simulink library "lib_transmission2"  (Simulink 10.1)
settings: Solver=VariableStepAuto  StartTime=0.0  StopTime=10.0  RelTol=1e-3
undefined symbols (not defined in the file or in its folder): cyc_mph, fc_map_spd, fc_max_trq, fc_spd_scale, fc_trq_scale, fd_inertia, fd_loss, fd_ratio, gb_gear_number_lookup, gb_gears_num, gb_inertia, gb_loss_const, gb_loss_input_spd_coeff, gb_loss_input_trq_coeff, gb_loss_output_spd_coeff, gb_loss_output_trq_coeff, gb_num_init, gb_ratio, gb_shift_delay, gb_spd_scale, gb_trq_scale, htc_inertia, htc_k_adv, htc_k_adv_coast, htc_lockup, htc_lockup_load, htc_lockup_spd, htc_lu_gear_range, htc_max_coast_tr, htc_min_coast_tr, htc_pump_loss_spd, htc_pump_loss_trq_lockup, htc_pump_loss_trq_unlock, htc_sr, htc_sr_coast, htc_tr, htc_tr_coast, htc_unlock_spd, mc_map_spd, mc_max_trq, mc_overtrq_factor, mc_spd_scale, mc_trq_scale, tc_loss, tc_mc_to_fc_ratio, tx_eff_map, tx_map_spd, tx_map_trq, tx_pg_r, tx_pg_s, tx_speed_dep, vc_clutch_bool, vc_idle_spd, vc_launch_spd, wh_radius
undefined symbols (not defined in the file): gb_dnshift_load, gb_dnshift_spd, gb_map_spd_out, gb_map_trq_in, gb_map_trq_out, gb_upshift_load, gb_upshift_spd, logFlag
libraries: lib_controls x1, lib_etc x1, lib_controls2 x1, lib_transmission x1
(part 13 of 17)

== system lib_transmission2/gearbox <gb>/gearbox model & interface/gearbox model/gearbox controller interface ==
  T_gb_out : Inport
  w_gb_out : Inport  Port=2
  eta_gb : Inport  Port=3
  enhancedToWorkspace1 : Subsystem  mask(enhancedToWorkspace){generalName=generalName, specificName=gear_ratio, logFlag=logFlag}
      mask prompts: generalName "General Name [char-evaluated]"; specificName "Specific Name [char-literal]"; logFlag "Enable flag (1=on,0=off)"
      mask help: A wrapper for the Simulink "To Workspace" block that allows you to evaluate the name of the variable to log to workspace. This is useful to avoid the double logging errors that occur when you pull in two library models that attempt to log to the same variable.
      mask init:
      | enhancedToWsMaker
      settings: CopyFcn=breakLinkCopyFcn  ParentCloseFcn=breakLinkParCloseFcn
      mask Help:
      | <h2>Enhanced To Workspace Block</h2>
      | <h3>Parameters</h3>
      | <UL>
      | <li><b>General Name:</b> This is the more general name of the variable. Variables are saved to the workspace as <i>generalName_specificName</i>. Note that this is an evaluated variable. If you would like to type in the value directly, it must be surrounded with single quotes. Otherwise you can input the name of a variable containing a char string.</li>
      | <li><b>Specific Name:</b> This is the specific name of the variable. Note that this is input as a char literal (i.e., you don't need quotes).</li>
      | <li><b>Enable Flag:</b> This flag should have the value of 0 or 1. If 0, the variable will not be logged to the workspace. If 1, the variable will be logged. This is done so that variable logging can be turned off to improve speed.</li>
      | </ul>
      | <h3>Overview</h3>
      | <p>The enhanced to workspace block was put together to allow one to dynamically resolve variable names at run time in simulink. This is most powerful when used in conjunction with a masked subsystem to allow multiple instances of that masked subsytem to be used in the same model. The strategy is to set the generalName in the block mask which will allow the block to change the general name for all variable logging on the fly.
      | <h3>Helper Files</h3>
      | <p>Three m-files are required by the enhancedToWorkspace block. These files are located in the &lt; ADVISOR root &gt;/GUI directory :
      | <ul>
      | <li><i>enhancedToWsMaker.m</i> This file runs the mask initialization for the block</li>
      | <li><i>breakLinkCopyFcn.m</i> This file is used by the block callback when the simulink block is copied. It is necessary to break the link to the enhancedToWorkspace similar to the To Workspace block in order for it to be able to configure itself. (Try copying simulink's To Workspace block--it is impossible to make a link)</li>
      | <li><i>breakLinkParCloseFcn.m</i> This file is similar to the breakLinkCopyFcn and is used when a parent system is closed</li>
      | </ul>
      | <hr>
      | 
      | <p>Created 2003-Jan-21, Michael Patrick O'Keefe, NREL</p>
      mask Display: disp([generalName,'_',specificName])
  enhancedToWorkspace8 : Subsystem  mask(enhancedToWorkspace){generalName=generalName, specificName=shifting, logFlag=logFlag}
      mask prompts: generalName "General Name [char-evaluated]"; specificName "Specific Name [char-literal]"; logFlag "Enable flag (1=on,0=off)"
      mask help: A wrapper for the Simulink "To Workspace" block that allows you to evaluate the name of the variable to log to workspace. This is useful to avoid the double logging errors that occur when you pull in two library models that attempt to log to the same variable.
      mask init:
      | enhancedToWsMaker
      settings: CopyFcn=breakLinkCopyFcn  ParentCloseFcn=breakLinkParCloseFcn
      mask Help:
      | <h2>Enhanced To Workspace Block</h2>
      | <h3>Parameters</h3>
      | <UL>
      | <li><b>General Name:</b> This is the more general name of the variable. Variables are saved to the workspace as <i>generalName_specificName</i>. Note that this is an evaluated variable. If you would like to type in the value directly, it must be surrounded with single quotes. Otherwise you can input the name of a variable containing a char string.</li>
      | <li><b>Specific Name:</b> This is the specific name of the variable. Note that this is input as a char literal (i.e., you don't need quotes).</li>
      | <li><b>Enable Flag:</b> This flag should have the value of 0 or 1. If 0, the variable will not be logged to the workspace. If 1, the variable will be logged. This is done so that variable logging can be turned off to improve speed.</li>
      | </ul>
      | <h3>Overview</h3>
      | <p>The enhanced to workspace block was put together to allow one to dynamically resolve variable names at run time in simulink. This is most powerful when used in conjunction with a masked subsystem to allow multiple instances of that masked subsytem to be used in the same model. The strategy is to set the generalName in the block mask which will allow the block to change the general name for all variable logging on the fly.
      | <h3>Helper Files</h3>
      | <p>Three m-files are required by the enhancedToWorkspace block. These files are located in the &lt; ADVISOR root &gt;/GUI directory :
      | <ul>
      | <li><i>enhancedToWsMaker.m</i> This file runs the mask initialization for the block</li>
      | <li><i>breakLinkCopyFcn.m</i> This file is used by the block callback when the simulink block is copied. It is necessary to break the link to the enhancedToWorkspace similar to the To Workspace block in order for it to be able to configure itself. (Try copying simulink's To Workspace block--it is impossible to make a link)</li>
      | <li><i>breakLinkParCloseFcn.m</i> This file is similar to the breakLinkCopyFcn and is used when a parent system is closed</li>
      | </ul>
      | <hr>
      | 
      | <p>Created 2003-Jan-21, Michael Patrick O'Keefe, NREL</p>
      mask Display: disp([generalName,'_',specificName])
  gear_ratio : Outport  InitialOutput=0
  shifting : Outport  Port=2  InitialOutput=0
  tag scope: T_gb_out=scoped, eta_gb=scoped, w_gb_out=scoped
  wires:
  [gear_ratio] -> gear_ratio/1, enhancedToWorkspace1/1(In1)
  eta_gb/1 -> [eta_gb]
  w_gb_out/1 -> [w_gb_out]
  T_gb_out/1 -> [T_gb_out]
  [shifting] -> shifting/1, enhancedToWorkspace8/1(In1)

== system lib_transmission2/gearbox <gb>/gearbox model & interface/gearbox model/gearing (Nm) (rad/s) ==
  "output shaft torque and speed  (Nm), (rad/s)" : Inport
  gear ratio : Inport  Port=2
  Demux : Demux  Outputs=2
  Fcn1 : Fcn  Expr=1/u
  Product2 : Product  SaturateOnIntegerOverflow=on
  Product3 : Product  SaturateOnIntegerOverflow=on
  input shaft torque (Nm) : Outport  InitialOutput=0
  input shaft speed (rad/s) : Outport  Port=2  InitialOutput=0
  wires:
  Product3/1 -> input shaft speed (rad/s)/1
  Product2/1 -> input shaft torque (Nm)/1
  Fcn1/1 -> Product2/2
  "output shaft torque and speed  (Nm), (rad/s)"/1 -> Demux/1
  gear ratio/1 -> Fcn1/1, Product3/2
  Demux/1 -> Product2/1
  Demux/2 -> Product3/1

== system lib_transmission2/gearbox <gb>/gearbox model & interface/gearbox model/gearing (Nm) (rad/s)1 ==
  input shaft torque (Nm) : Inport
  input shaft speed (rad/s) : Inport  Port=2
  gear ratio : Inport  Port=3
  Fcn1 : Fcn  Expr=1/u
  Product2 : Product  SaturateOnIntegerOverflow=on
  Product3 : Product  SaturateOnIntegerOverflow=on
  output shaft torque (Nm) : Outport  InitialOutput=0
  output shaft speed (rad/s) : Outport  Port=2  InitialOutput=0
  wires:
  Fcn1/1 -> Product3/1
  gear ratio/1 -> Product2/2, Fcn1/1
  Product3/1 -> output shaft speed (rad/s)/1
  Product2/1 -> output shaft torque (Nm)/1
  input shaft torque (Nm)/1 -> Product2/1
  input shaft speed (rad/s)/1 -> Product3/2

== system lib_transmission2/gearbox <gb>/gearbox model & interface/gearbox model/help ==

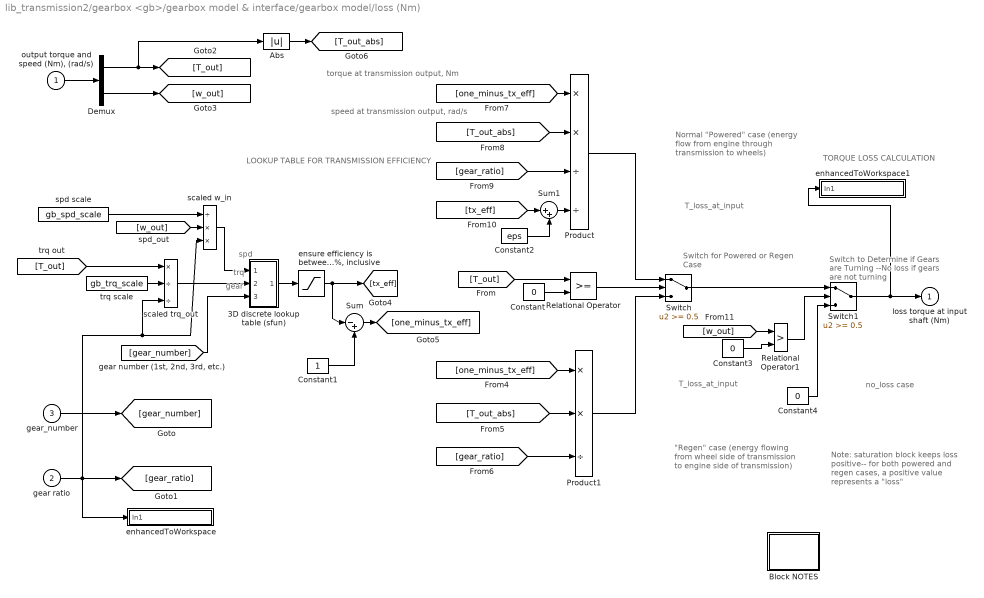
== system lib_transmission2/gearbox <gb>/gearbox model & interface/gearbox model/loss (Nm) ==
  note: TORQUE LOSS CALCULATION
  note: gear
  note: trq
  note: spd
  note: torque at transmission output, Nm
  note: speed at transmission output, rad/s
  note: no_loss case
  note: Note: saturation block keeps
      | loss positive-- for both powered
      | and regen cases, a
      | positive value represents a "loss"
  note: Switch for Powered
      |  or Regen Case
  note: Switch to Determine
      | if Gears are Turning
      | --No loss if gears
      | are not turning
  note: Normal "Powered" case
      | (energy flow from engine
      | through transmission to wheels)
  note: T_loss_at_input
  note: "Regen" case
      | (energy flowing from
      | wheel side of transmission
      | to engine side of transmission)
  note: T_loss_at_input
  note: LOOKUP TABLE FOR TRANSMISSION EFFICIENCY
  "output torque and speed (Nm), (rad/s)" : Inport
  gear ratio : Inport  Port=2
  gear_number : Inport  Port=3
  3D discrete lookup table (sfun) : Subsystem  AncestorBlock=|  mask{tx_map_spd=tx_map_spd, tx_map_trq=tx_map_trq, tx_eff_map=tx_eff_map}
      | lib_transmission/SubLibraries/3D discrete lookup
      | table (sfun)
      mask prompts: tx_map_spd "Row Lookup"; tx_map_trq "Column Lookup"; tx_eff_map "Lookup Matrix"
  Abs : Abs  SaturateOnIntegerOverflow=on
  Block NOTES : Subsystem
      mask Display: disp('Block\nNOTES')
  Constant : Constant  Value=0
  Constant1 : Constant
  Constant2 : Constant  Value=eps
  Constant3 : Constant  Value=0
  Constant4 : Constant  Value=0
  Demux : Demux  Outputs=2
  Product : Product  Inputs=**//  SaturateOnIntegerOverflow=on
  Product1 : Product  Inputs=**/  SaturateOnIntegerOverflow=on
  Relational Operator : RelationalOperator  RndMeth=Nearest  InputSameDT=on
  Relational Operator1 : RelationalOperator  Operator=>  RndMeth=Nearest  InputSameDT=on
  Sum : Sum  Inputs=|-+  SaturateOnIntegerOverflow=on
  Sum1 : Sum  Inputs=|++  SaturateOnIntegerOverflow=on
  Switch : Switch  Threshold=0.5  SaturateOnIntegerOverflow=on  InputSameDT=on
  Switch1 : Switch  Threshold=0.5  SaturateOnIntegerOverflow=on  InputSameDT=on
  enhancedToWorkspace : Subsystem  TreatAsAtomicUnit=on  mask(enhancedToWorkspace){generalName=generalName, specificName=current_gear_ratio, logFlag=logFlag}
      mask prompts: generalName "General Name [char-evaluated]"; specificName "Specific Name [char-literal]"; logFlag "Enable flag (1=on,0=off)"
      mask help: A wrapper for the Simulink "To Workspace" block that allows you to evaluate the name of the variable to log to workspace. This is useful to avoid the double logging errors that occur when you pull in two library models that attempt to log to the same variable.
      mask init:
      | enhancedToWsMaker
      settings: CopyFcn=breakLinkCopyFcn  ParentCloseFcn=breakLinkParCloseFcn
      mask Help:
      | <h2>Enhanced To Workspace Block</h2>
      | <h3>Parameters</h3>
      | <UL>
      | <li><b>General Name:</b> This is the more general name of the variable. Variables are saved to the workspace as <i>generalName_specificName</i>. Note that this is an evaluated variable. If you would like to type in the value directly, it must be surrounded with single quotes. Otherwise you can input the name of a variable containing a char string.</li>
      | <li><b>Specific Name:</b> This is the specific name of the variable. Note that this is input as a char literal (i.e., you don't need quotes).</li>
      | <li><b>Enable Flag:</b> This flag should have the value of 0 or 1. If 0, the variable will not be logged to the workspace. If 1, the variable will be logged. This is done so that variable logging can be turned off to improve speed.</li>
      | </ul>
      | <h3>Overview</h3>
      | <p>The enhanced to workspace block was put together to allow one to dynamically resolve variable names at run time in simulink. This is most powerful when used in conjunction with a masked subsystem to allow multiple instances of that masked subsytem to be used in the same model. The strategy is to set the generalName in the block mask which will allow the block to change the general name for all variable logging on the fly.
      | <h3>Helper Files</h3>
      | <p>Three m-files are required by the enhancedToWorkspace block. These files are located in the &lt; ADVISOR root &gt;/GUI directory :
      | <ul>
      | <li><i>enhancedToWsMaker.m</i> This file runs the mask initialization for the block</li>
      | <li><i>breakLinkCopyFcn.m</i> This file is used by the block callback when the simulink block is copied. It is necessary to break the link to the enhancedToWorkspace similar to the To Workspace block in order for it to be able to configure itself. (Try copying simulink's To Workspace block--it is impossible to make a link)</li>
      | <li><i>breakLinkParCloseFcn.m</i> This file is similar to the breakLinkCopyFcn and is used when a parent system is closed</li>
      | </ul>
      | <hr>
      | 
      | <p>Created 2003-Jan-21, Michael Patrick O'Keefe, NREL</p>
      | 
      | <!--
      | <VARDEF>
      | <H3>var_name</H3>
      | <UL>
      | <LI><B>data type</B> data type here</LI>
      | <LI><B>units</B> units here</LI>
      | <LI><B>vehicle type</B> vehicle type here</LI>
      | <LI><B>description</B> description here</LI>
      | </UL>
      | </VARDEF>
      | -->
      mask Display: disp([generalName,'_',specificName])
  enhancedToWorkspace1 : Subsystem  TreatAsAtomicUnit=on  mask(enhancedToWorkspace){generalName=generalName, specificName=spin_loss_trq, logFlag=logFlag}
      mask prompts: generalName "General Name [char-evaluated]"; specificName "Specific Name [char-literal]"; logFlag "Enable flag (1=on,0=off)"
      mask help: A wrapper for the Simulink "To Workspace" block that allows you to evaluate the name of the variable to log to workspace. This is useful to avoid the double logging errors that occur when you pull in two library models that attempt to log to the same variable.
      mask init:
      | enhancedToWsMaker
      settings: CopyFcn=breakLinkCopyFcn  ParentCloseFcn=breakLinkParCloseFcn
      mask Help:
      | <h2>Enhanced To Workspace Block</h2>
      | <h3>Parameters</h3>
      | <UL>
      | <li><b>General Name:</b> This is the more general name of the variable. Variables are saved to the workspace as <i>generalName_specificName</i>. Note that this is an evaluated variable. If you would like to type in the value directly, it must be surrounded with single quotes. Otherwise you can input the name of a variable containing a char string.</li>
      | <li><b>Specific Name:</b> This is the specific name of the variable. Note that this is input as a char literal (i.e., you don't need quotes).</li>
      | <li><b>Enable Flag:</b> This flag should have the value of 0 or 1. If 0, the variable will not be logged to the workspace. If 1, the variable will be logged. This is done so that variable logging can be turned off to improve speed.</li>
      | </ul>
      | <h3>Overview</h3>
      | <p>The enhanced to workspace block was put together to allow one to dynamically resolve variable names at run time in simulink. This is most powerful when used in conjunction with a masked subsystem to allow multiple instances of that masked subsytem to be used in the same model. The strategy is to set the generalName in the block mask which will allow the block to change the general name for all variable logging on the fly.
      | <h3>Helper Files</h3>
      | <p>Three m-files are required by the enhancedToWorkspace block. These files are located in the &lt; ADVISOR root &gt;/GUI directory :
      | <ul>
      | <li><i>enhancedToWsMaker.m</i> This file runs the mask initialization for the block</li>
      | <li><i>breakLinkCopyFcn.m</i> This file is used by the block callback when the simulink block is copied. It is necessary to break the link to the enhancedToWorkspace similar to the To Workspace block in order for it to be able to configure itself. (Try copying simulink's To Workspace block--it is impossible to make a link)</li>
      | <li><i>breakLinkParCloseFcn.m</i> This file is similar to the breakLinkCopyFcn and is used when a parent system is closed</li>
      | </ul>
      | <hr>
      | 
      | <p>Created 2003-Jan-21, Michael Patrick O'Keefe, NREL</p>
      | 
      | <!--
      | <VARDEF>
      | <H3>var_name</H3>
      | <UL>
      | <LI><B>data type</B> data type here</LI>
      | <LI><B>units</B> units here</LI>
      | <LI><B>vehicle type</B> vehicle type here</LI>
      | <LI><B>description</B> description here</LI>
      | </UL>
      | </VARDEF>
      | -->
      mask Display: disp([generalName,'_',specificName])
  "ensure efficiency is between  0% and 100%, inclusive" : Saturate  UpperLimit=1  LowerLimit=0
  scaled trq_out : Product  Inputs=*//  SaturateOnIntegerOverflow=on
  scaled w_in : Product  Inputs=/**  SaturateOnIntegerOverflow=on
  spd scale : Constant  Value=gb_spd_scale
  trq scale : Constant  Value=gb_trq_scale
  loss torque at input shaft (Nm) : Outport  InitialOutput=0
  wires:
  gear_number/1 -> [gear_number]
  gear ratio/1 -> [gear_ratio], scaled w_in/3, scaled trq_out/3, enhancedToWorkspace/1(In1)
  spd scale/1 -> scaled w_in/1
  [w_out] -> scaled w_in/2
  Sum/1 -> [one_minus_tx_eff]
  Constant1/1 -> Sum/2
  trq scale/1 -> scaled trq_out/2
  scaled trq_out/1 -> 3D discrete lookup table (sfun)/2(lookup trq (Nm))
  [T_out] -> scaled trq_out/1
  scaled w_in/1 -> 3D discrete lookup table (sfun)/1(lookup speed (rad/s))
  "ensure efficiency is between  0% and 100%, inclusive"/1 -> Sum/1, [tx_eff]
  3D discrete lookup table (sfun)/1(tx_eff) -> "ensure efficiency is between  0% and 100%, inclusive"/1
  Switch/1 -> Switch1/1
  Abs/1 -> [T_out_abs]
  Demux/1 -> Abs/1, [T_out]
  Relational Operator1/1 -> Switch1/2
  Constant3/1 -> Relational Operator1/2
  [w_out] -> Relational Operator1/1
  Constant4/1 -> Switch1/3
  Switch1/1 -> loss torque at input shaft (Nm)/1, enhancedToWorkspace1/1(In1)
  Constant2/1 -> Sum1/2
  [tx_eff] -> Sum1/1
  Sum1/1 -> Product/4
  [gear_ratio] -> Product/3
  [T_out_abs] -> Product/2
  [one_minus_tx_eff] -> Product/1
  Product/1 -> Switch/1
  [T_out_abs] -> Product1/2
  [gear_ratio] -> Product1/3
  [one_minus_tx_eff] -> Product1/1
  Product1/1 -> Switch/3
  [T_out] -> Relational Operator/1
  Constant/1 -> Relational Operator/2
  Relational Operator/1 -> Switch/2
  [gear_number] -> 3D discrete lookup table (sfun)/3("gear_number  (e.g., 1, 2, 3)")
  Demux/2 -> [w_out]
  "output torque and speed (Nm), (rad/s)"/1 -> Demux/1

== system lib_transmission2/gearbox <gb> CVT/CVT model & interface/CVT gearbox  <gb>/Block NOTES1 ==
  note: This gearbox model includes loss data, rotational inertia, and a gear reduction.
  note: The loss torque is zero when the gears are not turning,
      | and is applied at the input side of the gear reduction.
  note: The inertia torque is the input torque required to accelerate the
      | final drive's inertia as measured on the input side.
  note: Available output torque is estimated assuming that the gearbox efficiency for theavailable input
      | torque andspeed is the same as the gearbox efficiency for the REQUESTED input torque.
  note: This is a good assumption, at least for the VW 4-speed manual transaxle of SAE 820741.
      | In the VW transaxle, efficiency is fairly independent of torque and speed at high torques.

== system lib_transmission2/gearbox <gb> CVT/CVT model & interface/CVT gearbox  <gb>/Pout/Pin, neglecting inertia ==
  note: Pout/Pin, neglecting inertia, is used to estimate the output torque given the
      | input torque in a very simple forward-facing calculation.
  Tin : Inport
  Tinertia : Inport  Port=2
  Tout : Inport  Port=3
  gear ratio : Inport  Port=4
  Constant : Constant  Value=eps
  Constant2 : Constant  Value=0.5
  Pout/Pin (neglecting inertia) : Product  Inputs=*/  SaturateOnIntegerOverflow=on
  Product : Product  SaturateOnIntegerOverflow=on
  Switch : Switch  Threshold=eps  SaturateOnIntegerOverflow=on  InputSameDT=on
  Tin-Tinertia : Sum  Inputs=+-  SaturateOnIntegerOverflow=on
  make division bombproof : Sum  SaturateOnIntegerOverflow=on
  Pout/Pin : Outport  InitialOutput=0
  wires:
  Switch/1 -> Pout/Pin/1
  Pout/Pin (neglecting inertia)/1 -> Switch/2, Switch/1
  Product/1 -> Pout/Pin (neglecting inertia)/2
  Constant2/1 -> Switch/3
  gear ratio/1 -> Product/1
  make division bombproof/1 -> Product/2
  Tinertia/1 -> Tin-Tinertia/2
  Tout/1 -> Pout/Pin (neglecting inertia)/1
  Tin/1 -> Tin-Tinertia/1
  Tin-Tinertia/1 -> make division bombproof/1
  Constant/1 -> make division bombproof/2

== system lib_transmission2/gearbox <gb> CVT/CVT model & interface/CVT gearbox  <gb>/cvt controller interface ==
  T_gb_out : Inport
  w_gb_out : Inport  Port=2
  eta_gb : Inport  Port=3
  gear_ratio : Outport  InitialOutput=0
  tag scope: T_gb_out=global, eta_gb=global, w_gb_out=global
  wires:
  T_gb_out/1 -> [T_gb_out]
  w_gb_out/1 -> [w_gb_out]
  eta_gb/1 -> [eta_gb]
  [gear_ratio] -> gear_ratio/1

== system lib_transmission2/gearbox <gb> CVT/CVT model & interface/CVT gearbox  <gb>/effect of inertia (Nm) ==
  note: The inertia torque is the input torque required to accelerate the
      | gearbox's inertia as measured on the input side.
  gb input speed (rad/s) : Inport
  Gain : Gain  Gain=gb_inertia  SaturateOnIntegerOverflow=on
  d/dt : Derivative
  drag torque (Nm) : Outport  InitialOutput=0
  wires:
  Gain/1 -> drag torque (Nm)/1
  gb input speed (rad/s)/1 -> d/dt/1
  d/dt/1 -> Gain/1

== system lib_transmission2/gearbox <gb> CVT/CVT model & interface/CVT gearbox  <gb>/enhancedToWorkspace ==
  In1 : Inport
  Terminator : Terminator
  wires:
  In1/1 -> Terminator/1

== system lib_transmission2/gearbox <gb> CVT/CVT model & interface/CVT gearbox  <gb>/enhancedToWorkspace1 ==
  In1 : Inport
  Terminator : Terminator
  wires:
  In1/1 -> Terminator/1

== system lib_transmission2/gearbox <gb> CVT/CVT model & interface/CVT gearbox  <gb>/enhancedToWorkspace2 ==
  In1 : Inport
  Terminator : Terminator
  wires:
  In1/1 -> Terminator/1

== system lib_transmission2/gearbox <gb> CVT/CVT model & interface/CVT gearbox  <gb>/enhancedToWorkspace3 ==
  In1 : Inport
  Terminator : Terminator
  wires:
  In1/1 -> Terminator/1

== system lib_transmission2/gearbox <gb> CVT/CVT model & interface/CVT gearbox  <gb>/enhancedToWorkspace4 ==
  In1 : Inport
  Terminator : Terminator
  wires:
  In1/1 -> Terminator/1

== system lib_transmission2/gearbox <gb> CVT/CVT model & interface/CVT gearbox  <gb>/enhancedToWorkspace5 ==
  In1 : Inport
  Terminator : Terminator
  wires:
  In1/1 -> Terminator/1

== system lib_transmission2/gearbox <gb> CVT/CVT model & interface/CVT gearbox  <gb>/enhancedToWorkspace6 ==
  In1 : Inport
  Terminator : Terminator
  wires:
  In1/1 -> Terminator/1

== system lib_transmission2/gearbox <gb> CVT/CVT model & interface/CVT gearbox  <gb>/enhancedToWorkspace7 ==
  In1 : Inport
  Terminator : Terminator
  wires:
  In1/1 -> Terminator/1

== system lib_transmission2/gearbox <gb> CVT/CVT model & interface/CVT gearbox  <gb>/enhancedToWorkspace8 ==
  In1 : Inport
  Terminator : Terminator
  wires:
  In1/1 -> Terminator/1

== system lib_transmission2/gearbox <gb> CVT/CVT model & interface/CVT gearbox  <gb>/gearbox  efficiency ==
  In1 : Inport
  Constant : Constant  Value=eps
  Constant1 : Constant
  Product : Product  Inputs=*/  SaturateOnIntegerOverflow=on
  Switch : Switch  Threshold=1  SaturateOnIntegerOverflow=on  InputSameDT=on
  enhancedToWorkspace : Subsystem  TreatAsAtomicUnit=on  mask(enhancedToWorkspace){generalName=generalName, specificName=eta_gb, logFlag=logFlag}
      mask prompts: generalName "General Name [char-evaluated]"; specificName "Specific Name [char-literal]"; logFlag "Enable flag (1=on,0=off)"
      mask help: A wrapper for the Simulink "To Workspace" block that allows you to evaluate the name of the variable to log to workspace. This is useful to avoid the double logging errors that occur when you pull in two library models that attempt to log to the same variable.
      mask init:
      | enhancedToWsMaker
      settings: CopyFcn=breakLinkCopyFcn  ParentCloseFcn=breakLinkParCloseFcn
      mask Help:
      | <h2>Enhanced To Workspace Block</h2>
      | <h3>Parameters</h3>
      | <UL>
      | <li><b>General Name:</b> This is the more general name of the variable. Variables are saved to the workspace as <i>generalName_specificName</i>. Note that this is an evaluated variable. If you would like to type in the value directly, it must be surrounded with single quotes. Otherwise you can input the name of a variable containing a char string.</li>
      | <li><b>Specific Name:</b> This is the specific name of the variable. Note that this is input as a char literal (i.e., you don't need quotes).</li>
      | <li><b>Enable Flag:</b> This flag should have the value of 0 or 1. If 0, the variable will not be logged to the workspace. If 1, the variable will be logged. This is done so that variable logging can be turned off to improve speed.</li>
      | </ul>
      | <h3>Overview</h3>
      | <p>The enhanced to workspace block was put together to allow one to dynamically resolve variable names at run time in simulink. This is most powerful when used in conjunction with a masked subsystem to allow multiple instances of that masked subsytem to be used in the same model. The strategy is to set the generalName in the block mask which will allow the block to change the general name for all variable logging on the fly.
      | <h3>Helper Files</h3>
      | <p>Three m-files are required by the enhancedToWorkspace block. These files are located in the &lt; ADVISOR root &gt;/GUI directory :
      | <ul>
      | <li><i>enhancedToWsMaker.m</i> This file runs the mask initialization for the block</li>
      | <li><i>breakLinkCopyFcn.m</i> This file is used by the block callback when the simulink block is copied. It is necessary to break the link to the enhancedToWorkspace similar to the To Workspace block in order for it to be able to configure itself. (Try copying simulink's To Workspace block--it is impossible to make a link)</li>
      | <li><i>breakLinkParCloseFcn.m</i> This file is similar to the breakLinkCopyFcn and is used when a parent system is closed</li>
      | </ul>
      | <hr>
      | 
      | <p>Created 2003-Jan-21, Michael Patrick O'Keefe, NREL</p>
      | 
      | <!--
      | <VARDEF>
      | <H3>var_name</H3>
      | <UL>
      | <LI><B>data type</B> data type here</LI>
      | <LI><B>units</B> units here</LI>
      | <LI><B>vehicle type</B> vehicle type here</LI>
      | <LI><B>description</B> description here</LI>
      | </UL>
      | </VARDEF>
      | -->
      mask Display: disp([generalName,'_',specificName])
  make division bombproof : Sum  SaturateOnIntegerOverflow=on
  wires:
  Product/1 -> Switch/1
  Constant1/1 -> Product/1
  make division bombproof/1 -> Product/2
  In1/1 -> Switch/3, Switch/2, make division bombproof/1
  Switch/1 -> enhancedToWorkspace/1(In1)
  Constant/1 -> make division bombproof/2

== system lib_transmission2/gearbox <gb> CVT/CVT model & interface/CVT gearbox  <gb>/gearing (Nm), (rad/s) ==
  "output shaft torque and speed  (Nm), (rad/s)" : Inport
  gear ratio : Inport  Port=2
  Demux : Demux  Outputs=2
  Fcn1 : Fcn  Expr=1/u
  Product2 : Product  SaturateOnIntegerOverflow=on
  Product3 : Product  SaturateOnIntegerOverflow=on
  input shaft torque (Nm) : Outport  InitialOutput=0
  input shaft speed (rad/s) : Outport  Port=2  InitialOutput=0
  wires:
  Product3/1 -> input shaft speed (rad/s)/1
  Product2/1 -> input shaft torque (Nm)/1
  Fcn1/1 -> Product2/2
  "output shaft torque and speed  (Nm), (rad/s)"/1 -> Demux/1
  gear ratio/1 -> Fcn1/1, Product3/2
  Demux/1 -> Product2/1
  Demux/2 -> Product3/1

== system lib_transmission2/gearbox <gb> CVT/CVT model & interface/CVT gearbox  <gb>/gearing (Nm), (rad/s)1 ==
  input shaft torque (Nm) : Inport
  input shaft speed (rad/s) : Inport  Port=2
  gear ratio : Inport  Port=3
  Fcn1 : Fcn  Expr=1/u
  Product2 : Product  SaturateOnIntegerOverflow=on
  Product3 : Product  SaturateOnIntegerOverflow=on
  output shaft torque (Nm) : Outport  InitialOutput=0
  output shaft speed (rad/s) : Outport  Port=2  InitialOutput=0
  wires:
  input shaft speed (rad/s)/1 -> Product3/2
  input shaft torque (Nm)/1 -> Product2/1
  Product2/1 -> output shaft torque (Nm)/1
  Product3/1 -> output shaft speed (rad/s)/1
  gear ratio/1 -> Fcn1/1, Product2/2
  Fcn1/1 -> Product3/1

== system lib_transmission2/gearbox <gb> CVT/CVT model & interface/CVT gearbox  <gb>/help1 ==

== system lib_transmission2/gearbox <gb> CVT/CVT model & interface/CVT gearbox  <gb>/loss (Nm) ==
  "output torque and speed (Nm), (rad/s)" : Inport
  pulley ratio : Inport  Port=2
  Abs2 : Abs  SaturateOnIntegerOverflow=on
  Demux1 : Demux  Outputs=2
  Input Torque: 3-D interpolation : Subsystem
  Product3 : Product  Inputs=*/  SaturateOnIntegerOverflow=on
  Sum2 : Sum  Inputs=-+  SaturateOnIntegerOverflow=on
  loss torque at input shaft (Nm) : Outport  InitialOutput=0
  wires:
  Demux1/2 -> Input Torque: 3-D interpolation/2(output speed (rad/s))
  "output torque and speed (Nm), (rad/s)"/1 -> Demux1/1
  pulley ratio/1 -> Input Torque: 3-D interpolation/3(pulley ratio), Product3/2
  Demux1/1 -> Input Torque: 3-D interpolation/1(output torque (N*m)), Product3/1
  Product3/1 -> Sum2/1
  Sum2/1 -> Abs2/1
  Abs2/1 -> loss torque at input shaft (Nm)/1
  Input Torque: 3-D interpolation/1(input torque (Nm)) -> Sum2/2

== system lib_transmission2/gearbox <gb> old/gearbox model & interface/gearbox model/Block NOTES ==
  note: This gearbox model includes loss data, rotational inertia, and a gear reduction.
  note: The loss torque is zero when the gears are not turning,
      | and is applied at the input side of the gear reduction.
  note: The inertia torque is the input torque required to accelerate the
      | final drive's inertia as measured on the input side.
  note: Available output torque is estimated assuming that the gearbox efficiency for theavailable input
      | torque andspeed is the same as the gearbox efficiency for the REQUESTED input torque.
  note: This is a good assumption, at least for the VW 4-speed manual transaxle of SAE 820741.
      | In the VW transaxle, efficiency is fairly independent of torque and speed at high torques.

== system lib_transmission2/gearbox <gb> old/gearbox model & interface/gearbox model/Pout/Pin neglecting inertia ==
  note: Pout/Pin, neglecting inertia, is used to estimate the output torque given the
      | input torque in a very simple forward-facing calculation.
  Tin : Inport
  Tinertia : Inport  Port=2
  Tout : Inport  Port=3
  gear ratio : Inport  Port=4
  Constant1 : Constant  Value=0
  Pout/Pin (neglecting inertia) : Subsystem
      mask Display: disp('/')
  Product : Product  SaturateOnIntegerOverflow=on
  Relational Operator : RelationalOperator  Operator=~=  RndMeth=Nearest  InputSameDT=on
  Saturation : Saturate  UpperLimit=inf  LowerLimit=0
  Switch : Switch  Threshold=eps  SaturateOnIntegerOverflow=on  InputSameDT=on
  Tin-Tinertia : Sum  Inputs=+-  SaturateOnIntegerOverflow=on
  make division bombproof : Subsystem
  Pout/Pin : Outport  InitialOutput=0
  wires:
  Constant1/1 -> Switch/3, Relational Operator/2
  make division bombproof/1(Out1) -> Product/2
  Tinertia/1 -> Tin-Tinertia/2
  Tin/1 -> Tin-Tinertia/1
  Pout/Pin (neglecting inertia)/1(out_1) -> Switch/1
  Relational Operator/1 -> Switch/2
  Switch/1 -> Saturation/1
  Saturation/1 -> Pout/Pin/1
  Tin-Tinertia/1 -> Relational Operator/1, make division bombproof/1(Tin-Tinertia)
  Tout/1 -> Pout/Pin (neglecting inertia)/1(in_1)
  Product/1 -> Pout/Pin (neglecting inertia)/2(in_2)
  gear ratio/1 -> Product/1

== system lib_transmission2/gearbox <gb> old/gearbox model & interface/gearbox model/effect of inertia (Nm) ==
  note: The inertia torque is the input torque required to accelerate the
      | gearbox's inertia as measured on the input side.
  gb input speed (rad/s) : Inport
  Gain : Gain  Gain=gb_inertia  SaturateOnIntegerOverflow=on
  d/dt : Derivative
  drag torque (Nm) : Outport  InitialOutput=0
  wires:
  Gain/1 -> drag torque (Nm)/1
  d/dt/1 -> Gain/1
  gb input speed (rad/s)/1 -> d/dt/1

== system lib_transmission2/gearbox <gb> old/gearbox model & interface/gearbox model/enhancedToWorkspace ==
  In1 : Inport
  To Workspace : ToWorkspace  VariableName=gb_spd_in_a  SampleTime=-1
  wires:
  In1/1 -> To Workspace/1

== system lib_transmission2/gearbox <gb> old/gearbox model & interface/gearbox model/enhancedToWorkspace1 ==
  In1 : Inport
  To Workspace : ToWorkspace  VariableName=gb_trq_in_a  SampleTime=-1
  wires:
  In1/1 -> To Workspace/1

== system lib_transmission2/gearbox <gb> old/gearbox model & interface/gearbox model/enhancedToWorkspace2 ==
  In1 : Inport
  To Workspace : ToWorkspace  VariableName=gb_spd_out_a  SampleTime=-1
  wires:
  In1/1 -> To Workspace/1

== system lib_transmission2/gearbox <gb> old/gearbox model & interface/gearbox model/enhancedToWorkspace3 ==
  In1 : Inport
  To Workspace : ToWorkspace  VariableName=gb_trq_out_a  SampleTime=-1
  wires:
  In1/1 -> To Workspace/1

== system lib_transmission2/gearbox <gb> old/gearbox model & interface/gearbox model/enhancedToWorkspace4 ==
  In1 : Inport
  To Workspace : ToWorkspace  VariableName=gb_ni_trq_out_a  SampleTime=-1
  wires:
  In1/1 -> To Workspace/1

== system lib_transmission2/gearbox <gb> old/gearbox model & interface/gearbox model/enhancedToWorkspace5 ==
  In1 : Inport
  To Workspace : ToWorkspace  VariableName=gb_spd_in_r  SampleTime=-1
  wires:
  In1/1 -> To Workspace/1

== system lib_transmission2/gearbox <gb> old/gearbox model & interface/gearbox model/enhancedToWorkspace6 ==
  In1 : Inport
  To Workspace : ToWorkspace  VariableName=gb_trq_in_r  SampleTime=-1
  wires:
  In1/1 -> To Workspace/1

== system lib_transmission2/gearbox <gb> old/gearbox model & interface/gearbox model/enhancedToWorkspace7 ==
  In1 : Inport
  To Workspace : ToWorkspace  VariableName=gb_spd_out_r  SampleTime=-1
  wires:
  In1/1 -> To Workspace/1

== system lib_transmission2/gearbox <gb> old/gearbox model & interface/gearbox model/enhancedToWorkspace8 ==
  In1 : Inport
  To Workspace : ToWorkspace  VariableName=gb_trq_out_r  SampleTime=-1
  wires:
  In1/1 -> To Workspace/1

== system lib_transmission2/gearbox <gb> old/gearbox model & interface/gearbox model/enhancedToWorkspace9 ==
  In1 : Inport
  To Workspace : ToWorkspace  VariableName=gb_gear_number  SampleTime=-1
  wires:
  In1/1 -> To Workspace/1

== system lib_transmission2/gearbox <gb> old/gearbox model & interface/gearbox model/gearbox controller interface ==
  T_gb_out : Inport
  w_gb_out : Inport  Port=2
  eta_gb : Inport  Port=3
  enhancedToWorkspace1 : Subsystem  mask(enhancedToWorkspace){generalName=generalName, specificName=gear_ratio, logFlag=logFlag}
      mask prompts: generalName "General Name [char-evaluated]"; specificName "Specific Name [char-literal]"; logFlag "Enable flag (1=on,0=off)"
      mask help: A wrapper for the Simulink "To Workspace" block that allows you to evaluate the name of the variable to log to workspace. This is useful to avoid the double logging errors that occur when you pull in two library models that attempt to log to the same variable.
      mask init:
      | enhancedToWsMaker
      settings: CopyFcn=breakLinkCopyFcn  ParentCloseFcn=breakLinkParCloseFcn
      mask Help:
      | <h2>Enhanced To Workspace Block</h2>
      | <h3>Parameters</h3>
      | <UL>
      | <li><b>General Name:</b> This is the more general name of the variable. Variables are saved to the workspace as <i>generalName_specificName</i>. Note that this is an evaluated variable. If you would like to type in the value directly, it must be surrounded with single quotes. Otherwise you can input the name of a variable containing a char string.</li>
      | <li><b>Specific Name:</b> This is the specific name of the variable. Note that this is input as a char literal (i.e., you don't need quotes).</li>
      | <li><b>Enable Flag:</b> This flag should have the value of 0 or 1. If 0, the variable will not be logged to the workspace. If 1, the variable will be logged. This is done so that variable logging can be turned off to improve speed.</li>
      | </ul>
      | <h3>Overview</h3>
      | <p>The enhanced to workspace block was put together to allow one to dynamically resolve variable names at run time in simulink. This is most powerful when used in conjunction with a masked subsystem to allow multiple instances of that masked subsytem to be used in the same model. The strategy is to set the generalName in the block mask which will allow the block to change the general name for all variable logging on the fly.
      | <h3>Helper Files</h3>
      | <p>Three m-files are required by the enhancedToWorkspace block. These files are located in the &lt; ADVISOR root &gt;/GUI directory :
      | <ul>
      | <li><i>enhancedToWsMaker.m</i> This file runs the mask initialization for the block</li>
      | <li><i>breakLinkCopyFcn.m</i> This file is used by the block callback when the simulink block is copied. It is necessary to break the link to the enhancedToWorkspace similar to the To Workspace block in order for it to be able to configure itself. (Try copying simulink's To Workspace block--it is impossible to make a link)</li>
      | <li><i>breakLinkParCloseFcn.m</i> This file is similar to the breakLinkCopyFcn and is used when a parent system is closed</li>
      | </ul>
      | <hr>
      | 
      | <p>Created 2003-Jan-21, Michael Patrick O'Keefe, NREL</p>
      mask Display: disp([generalName,'_',specificName])
  enhancedToWorkspace8 : Subsystem  mask(enhancedToWorkspace){generalName=generalName, specificName=shifting, logFlag=logFlag}
      mask prompts: generalName "General Name [char-evaluated]"; specificName "Specific Name [char-literal]"; logFlag "Enable flag (1=on,0=off)"
      mask help: A wrapper for the Simulink "To Workspace" block that allows you to evaluate the name of the variable to log to workspace. This is useful to avoid the double logging errors that occur when you pull in two library models that attempt to log to the same variable.
      mask init:
      | enhancedToWsMaker
      settings: CopyFcn=breakLinkCopyFcn  ParentCloseFcn=breakLinkParCloseFcn
      mask Help:
      | <h2>Enhanced To Workspace Block</h2>
      | <h3>Parameters</h3>
      | <UL>
      | <li><b>General Name:</b> This is the more general name of the variable. Variables are saved to the workspace as <i>generalName_specificName</i>. Note that this is an evaluated variable. If you would like to type in the value directly, it must be surrounded with single quotes. Otherwise you can input the name of a variable containing a char string.</li>
      | <li><b>Specific Name:</b> This is the specific name of the variable. Note that this is input as a char literal (i.e., you don't need quotes).</li>
      | <li><b>Enable Flag:</b> This flag should have the value of 0 or 1. If 0, the variable will not be logged to the workspace. If 1, the variable will be logged. This is done so that variable logging can be turned off to improve speed.</li>
      | </ul>
      | <h3>Overview</h3>
      | <p>The enhanced to workspace block was put together to allow one to dynamically resolve variable names at run time in simulink. This is most powerful when used in conjunction with a masked subsystem to allow multiple instances of that masked subsytem to be used in the same model. The strategy is to set the generalName in the block mask which will allow the block to change the general name for all variable logging on the fly.
      | <h3>Helper Files</h3>
      | <p>Three m-files are required by the enhancedToWorkspace block. These files are located in the &lt; ADVISOR root &gt;/GUI directory :
      | <ul>
      | <li><i>enhancedToWsMaker.m</i> This file runs the mask initialization for the block</li>
      | <li><i>breakLinkCopyFcn.m</i> This file is used by the block callback when the simulink block is copied. It is necessary to break the link to the enhancedToWorkspace similar to the To Workspace block in order for it to be able to configure itself. (Try copying simulink's To Workspace block--it is impossible to make a link)</li>
      | <li><i>breakLinkParCloseFcn.m</i> This file is similar to the breakLinkCopyFcn and is used when a parent system is closed</li>
      | </ul>
      | <hr>
      | 
      | <p>Created 2003-Jan-21, Michael Patrick O'Keefe, NREL</p>
      mask Display: disp([generalName,'_',specificName])
  gear_ratio : Outport  InitialOutput=0
  shifting : Outport  Port=2  InitialOutput=0
  tag scope: T_gb_out=scoped, eta_gb=scoped, w_gb_out=scoped
  wires:
  [gear_ratio] -> gear_ratio/1, enhancedToWorkspace1/1(In1)
  eta_gb/1 -> [eta_gb]
  w_gb_out/1 -> [w_gb_out]
  T_gb_out/1 -> [T_gb_out]
  [shifting] -> shifting/1, enhancedToWorkspace8/1(In1)

== system lib_transmission2/gearbox <gb> old/gearbox model & interface/gearbox model/gearing (Nm) (rad/s) ==
  "output shaft torque and speed  (Nm), (rad/s)" : Inport
  gear ratio : Inport  Port=2
  Demux : Demux  Outputs=2
  Fcn1 : Fcn  Expr=1/u
  Product2 : Product  SaturateOnIntegerOverflow=on
  Product3 : Product  SaturateOnIntegerOverflow=on
  input shaft torque (Nm) : Outport  InitialOutput=0
  input shaft speed (rad/s) : Outport  Port=2  InitialOutput=0
  wires:
  Product3/1 -> input shaft speed (rad/s)/1
  Product2/1 -> input shaft torque (Nm)/1
  Fcn1/1 -> Product2/2
  "output shaft torque and speed  (Nm), (rad/s)"/1 -> Demux/1
  gear ratio/1 -> Fcn1/1, Product3/2
  Demux/1 -> Product2/1
  Demux/2 -> Product3/1

== system lib_transmission2/gearbox <gb> old/gearbox model & interface/gearbox model/gearing (Nm) (rad/s)1 ==
  input shaft torque (Nm) : Inport
  input shaft speed (rad/s) : Inport  Port=2
  gear ratio : Inport  Port=3
  Fcn1 : Fcn  Expr=1/u
  Product2 : Product  SaturateOnIntegerOverflow=on
  Product3 : Product  SaturateOnIntegerOverflow=on
  output shaft torque (Nm) : Outport  InitialOutput=0
  output shaft speed (rad/s) : Outport  Port=2  InitialOutput=0
  wires:
  Fcn1/1 -> Product3/1
  gear ratio/1 -> Product2/2, Fcn1/1
  Product3/1 -> output shaft speed (rad/s)/1
  Product2/1 -> output shaft torque (Nm)/1
  input shaft torque (Nm)/1 -> Product2/1
  input shaft speed (rad/s)/1 -> Product3/2

== system lib_transmission2/gearbox <gb> old/gearbox model & interface/gearbox model/help ==
